simulink model "c00014M_harness"  (R2018a)
settings: Solver=ode3  StartTime=0.0  StopTime=10.0  RelTol=1e-3  EnableMultiTasking=on
undefined symbols (not defined in the file): b, DiscIntNeverNeededParam, J, K, L, PosMinimaW4, R, sigbuilder_block
(part 1 of 8)
settings Model: Creator=aarrieta  LastModifiedBy=umarkiegi
settings DataIOCC: LimitDataPoints=on  SaveFormat=Array
settings OptimizationCC: LifeSpan=inf
settings DebuggingCC: UnderspecifiedInitializationDetection=Classic  MergeDetectMultiDrivingBlocksExec=none  SolverPrmCheckMsg=warning  StateNameClashWarn=warning  SFUnexpectedBacktrackingDiag=warning  SFNoUnconditionalDefaultTransitionDiag=warning  SFExecutionAtInitializationDiag=none
settings HardwareCC: ProdBitPerPointer=32  ProdBitPerSizeT=32  ProdBitPerPtrDiffT=32  ProdLargestAtomicFloat=None  ProdIntDivRoundTo=Undefined  ProdEndianess=Unspecified  ProdWordSize=32  ProdHWDeviceType=32-bit Generic
settings ModelReferenceCC: PropagateSignalLabelsOutOfModel=off
settings CodeAppCC: StateflowObjectComments=on
settings GRTTargetCC: TargetLangStandard=C89/C90 (ANSI)  GeneratePreprocessorConditionals=Disable all
settings ConfigComp: CovMetricSettings=dw  CovHtmlReporting=on  CovSaveCumulativeToWorkspaceVar=on  CovSaveSingleToWorkspaceVar=on  CovExternalEMLEnable=off  DVMaxTestCaseSteps=20  DVTestSuiteOptimization=CombinedObjectives (Nonlinear Extended)  DVDetectFloatOverflow=off

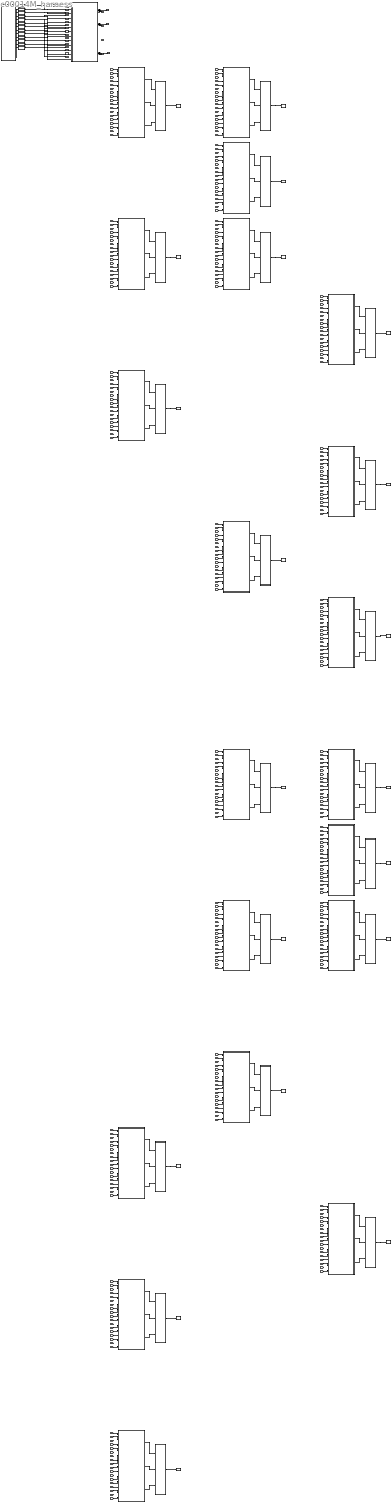
== system c00014M_harness ==
  CPSUT : Subsystem
  Eval : Subsystem
  Eval14 : Subsystem
  Eval16 : Subsystem
  Eval18 : Subsystem
  Eval2 : Subsystem
  Eval20 : Subsystem
  Eval21 : Subsystem
  Eval22 : Subsystem
  Eval26 : Subsystem
  Eval29 : Subsystem
  Eval31 : Subsystem
  Eval33 : Subsystem
  Eval4 : Subsystem
  Eval43 : Subsystem
  Eval45 : Subsystem
  Eval47 : Subsystem
  Eval49 : Subsystem
  Eval50 : Subsystem
  Eval51 : Subsystem
  Eval55 : Subsystem
  Inputs : Subsystem  Tag=STV Subsys  LoadFcn=sigbuilder_block('load');  StartFcn=sigbuilder_block('start');  StopFcn=sigbuilder_block('stop');  ClipboardFcn=sigbuilder_block('clipboard');  mask(Sigbuilder block){tuvar=[0:10]}
      mask init:
      | if ~strcmp(get_param(bdroot(gcb),'SimulationStatus'),'stopped'),tuvar = sigbuilder_block('maskInit'); end
      settings: CopyFcn=sigbuilder_block('copy');  DeleteFcn=sigbuilder_block('delete');  ModelCloseFcn=sigbuilder_block('modelClose');  PreSaveFcn=sigbuilder_block('preSave');  PauseFcn=sigbuilder_block('pause');  ContinueFcn=sigbuilder_block('continue');  NameChangeFcn=sigbuilder_block('namechange');  OpenFcn=sigbuilder_block('open');  CloseFcn=sigbuilder_block('close');
      mask Display: plot(0, 0, 100, 100,[2, 2, 32, 32, 2], [68, 8, 8, 68, 68],[32, 2], [38, 38], [32, 19, 2],[53, 60, 44], [32, 17, 17, 2],[16, 16, 31, 31]);txt = getActiveGroup(gcbh);text(2, 100, txt,'verticalAlignment', 'top');
  M001 : Subsystem
  M003 : Subsystem
  M005 : Subsystem
  M015 : Subsystem
  M017 : Subsystem
  M019 : Subsystem
  M021 : Subsystem
  M022 : Subsystem
  M023 : Subsystem
  M027 : Subsystem
  M030 : Subsystem
  M032 : Subsystem
  M034 : Subsystem
  M044 : Subsystem
  M046 : Subsystem
  M048 : Subsystem
  M050 : Subsystem
  M051 : Subsystem
  M052 : Subsystem
  M056 : Subsystem
  To Workspace : ToWorkspace  VariableName=mutant001  SampleTime=-1
  To Workspace14 : ToWorkspace  VariableName=mutant015  SampleTime=-1
  To Workspace16 : ToWorkspace  VariableName=mutant017  SampleTime=-1
  To Workspace18 : ToWorkspace  VariableName=mutant019  SampleTime=-1
  To Workspace2 : ToWorkspace  VariableName=mutant003  SampleTime=-1
  To Workspace20 : ToWorkspace  VariableName=mutant021  SampleTime=-1
  To Workspace21 : ToWorkspace  VariableName=mutant022  SampleTime=-1
  To Workspace22 : ToWorkspace  VariableName=mutant023  SampleTime=-1
  To Workspace26 : ToWorkspace  VariableName=mutant027  SampleTime=-1
  To Workspace29 : ToWorkspace  VariableName=mutant030  SampleTime=-1
  To Workspace31 : ToWorkspace  VariableName=mutant032  SampleTime=-1
  To Workspace33 : ToWorkspace  VariableName=mutant034  SampleTime=-1
  To Workspace4 : ToWorkspace  VariableName=mutant005  SampleTime=-1
  To Workspace43 : ToWorkspace  VariableName=mutant044  SampleTime=-1
  To Workspace45 : ToWorkspace  VariableName=mutant046  SampleTime=-1
  To Workspace47 : ToWorkspace  VariableName=mutant048  SampleTime=-1
  To Workspace49 : ToWorkspace  VariableName=mutant050  SampleTime=-1
  To Workspace50 : ToWorkspace  VariableName=mutant051  SampleTime=-1
  To Workspace51 : ToWorkspace  VariableName=mutant052  SampleTime=-1
  To Workspace55 : ToWorkspace  VariableName=mutant056  SampleTime=-1
  dtc_CW1C : DataTypeConversion
  dtc_CW2C : DataTypeConversion
  dtc_CW4C : DataTypeConversion
  dtc_DW1 : DataTypeConversion
  dtc_DW2 : DataTypeConversion
  dtc_DW4 : DataTypeConversion
  dtc_LD : DataTypeConversion
  dtc_O1 : DataTypeConversion
  dtc_O2 : DataTypeConversion
  dtc_O4 : DataTypeConversion
  dtc_P1W2 : DataTypeConversion
  dtc_P1W4 : DataTypeConversion
  dtc_P3W4 : DataTypeConversion
  W1Pos : Outport
  W2Pos : Outport  Port=2
  W4Pos : Outport  Port=3
  tag scope: out1=global, out2=global, out3=global, out4=global
  wires:
  CPSUT/2(W2Pos) -> [out2], W2Pos/1
  CPSUT/3(W4Pos) -> W4Pos/1, [out4]
  [in1] -> M001/1(DW1)
  [in2] -> M001/2(DW2)
  [in4] -> M001/3(DW4)
  [in5] -> M001/4(P1W2)
  [in8] -> M001/5(P3W4)
  [in9] -> M001/6(P1W4)
  [in10] -> M001/7(O1)
  [in11] -> M001/8(O2)
  [in13] -> M001/9(O4)
  [in14] -> M001/10(LD)
  [in15] -> M001/11(CW1C)
  [in16] -> M001/12(CW2C)
  [in18] -> M001/13(CW4C)
  CPSUT/1(W1Pos) -> [out1], W1Pos/1
  M001/1(W1Pos) -> Eval/1(In1)
  M001/2(W2Pos) -> Eval/2(In2)
  M001/3(W4Pos) -> Eval/3(In4)
  Eval/1(Out1) -> To Workspace/1
  [in1] -> M003/1(DW1)
  [in2] -> M003/2(DW2)
  [in4] -> M003/3(DW4)
  [in5] -> M003/4(P1W2)
  [in8] -> M003/5(P3W4)
  [in9] -> M003/6(P1W4)
  [in10] -> M003/7(O1)
  [in11] -> M003/8(O2)
  [in13] -> M003/9(O4)
  [in14] -> M003/10(LD)
  [in15] -> M003/11(CW1C)
  [in16] -> M003/12(CW2C)
  [in18] -> M003/13(CW4C)
  M003/1(W1Pos) -> Eval2/1(In1)
  M003/2(W2Pos) -> Eval2/2(In2)
  M003/3(W4Pos) -> Eval2/3(In4)
  Eval2/1(Out1) -> To Workspace2/1
  [in1] -> M005/1(DW1)
  [in2] -> M005/2(DW2)
  [in4] -> M005/3(DW4)
  [in5] -> M005/4(P1W2)
  [in8] -> M005/5(P3W4)
  [in9] -> M005/6(P1W4)
  [in10] -> M005/7(O1)
  [in11] -> M005/8(O2)
  [in13] -> M005/9(O4)
  [in14] -> M005/10(LD)
  [in15] -> M005/11(CW1C)
  [in16] -> M005/12(CW2C)
  [in18] -> M005/13(CW4C)
  M005/1(W1Pos) -> Eval4/1(In1)
  M005/2(W2Pos) -> Eval4/2(In2)
  M005/3(W4Pos) -> Eval4/3(In4)
  Eval4/1(Out1) -> To Workspace4/1
  [in1] -> M015/1(DW1)
  [in2] -> M015/2(DW2)
  [in4] -> M015/3(DW4)
  [in5] -> M015/4(P1W2)
  [in8] -> M015/5(P3W4)
  [in9] -> M015/6(P1W4)
  [in10] -> M015/7(O1)
  [in11] -> M015/8(O2)
  [in13] -> M015/9(O4)
  [in14] -> M015/10(LD)
  [in15] -> M015/11(CW1C)
  [in16] -> M015/12(CW2C)
  [in18] -> M015/13(CW4C)
  M015/1(W1Pos) -> Eval14/1(In1)
  M015/2(W2Pos) -> Eval14/2(In2)
  M015/3(W4Pos) -> Eval14/3(In4)
  Eval14/1(Out1) -> To Workspace14/1
  [in1] -> M017/1(DW1)
  [in2] -> M017/2(DW2)
  [in4] -> M017/3(DW4)
  [in5] -> M017/4(P1W2)
  [in8] -> M017/5(P3W4)
  [in9] -> M017/6(P1W4)
  [in10] -> M017/7(O1)
  [in11] -> M017/8(O2)
  [in13] -> M017/9(O4)
  [in14] -> M017/10(LD)
  [in15] -> M017/11(CW1C)
  [in16] -> M017/12(CW2C)
  [in18] -> M017/13(CW4C)
  M017/1(W1Pos) -> Eval16/1(In1)
  M017/2(W2Pos) -> Eval16/2(In2)
  M017/3(W4Pos) -> Eval16/3(In4)
  Eval16/1(Out1) -> To Workspace16/1
  [in1] -> M019/1(DW1)
  [in2] -> M019/2(DW2)
  [in4] -> M019/3(DW4)
  [in5] -> M019/4(P1W2)
  [in8] -> M019/5(P3W4)
  [in9] -> M019/6(P1W4)
  [in10] -> M019/7(O1)
  [in11] -> M019/8(O2)
  [in13] -> M019/9(O4)
  [in14] -> M019/10(LD)
  [in15] -> M019/11(CW1C)
  [in16] -> M019/12(CW2C)
  [in18] -> M019/13(CW4C)
  M019/1(W1Pos) -> Eval18/1(In1)
  M019/2(W2Pos) -> Eval18/2(In2)
  M019/3(W4Pos) -> Eval18/3(In4)
  Eval18/1(Out1) -> To Workspace18/1
  [in1] -> M021/1(DW1)
  [in2] -> M021/2(DW2)
  [in4] -> M021/3(DW4)
  [in5] -> M021/4(P1W2)
  [in8] -> M021/5(P3W4)
  [in9] -> M021/6(P1W4)
  [in10] -> M021/7(O1)
  [in11] -> M021/8(O2)
  [in13] -> M021/9(O4)
  [in14] -> M021/10(LD)
  [in15] -> M021/11(CW1C)
  [in16] -> M021/12(CW2C)
  [in18] -> M021/13(CW4C)
  M021/1(W1Pos) -> Eval20/1(In1)
  M021/2(W2Pos) -> Eval20/2(In2)
  M021/3(W4Pos) -> Eval20/3(In4)
  Eval20/1(Out1) -> To Workspace20/1
  [in1] -> M022/1(DW1)
  [in2] -> M022/2(DW2)
  [in4] -> M022/3(DW4)
  [in5] -> M022/4(P1W2)
  [in8] -> M022/5(P3W4)
  [in9] -> M022/6(P1W4)
  [in10] -> M022/7(O1)
  [in11] -> M022/8(O2)
  [in13] -> M022/9(O4)
  [in14] -> M022/10(LD)
  [in15] -> M022/11(CW1C)
  [in16] -> M022/12(CW2C)
  [in18] -> M022/13(CW4C)
  M022/1(W1Pos) -> Eval21/1(In1)
  M022/2(W2Pos) -> Eval21/2(In2)
  M022/3(W4Pos) -> Eval21/3(In4)
  Eval21/1(Out1) -> To Workspace21/1
  [in1] -> M023/1(DW1)
  [in2] -> M023/2(DW2)
  [in4] -> M023/3(DW4)
  [in5] -> M023/4(P1W2)
  [in8] -> M023/5(P3W4)
  [in9] -> M023/6(P1W4)
  [in10] -> M023/7(O1)
  [in11] -> M023/8(O2)
  [in13] -> M023/9(O4)
  [in14] -> M023/10(LD)
  [in15] -> M023/11(CW1C)
  [in16] -> M023/12(CW2C)
  [in18] -> M023/13(CW4C)
  M023/1(W1Pos) -> Eval22/1(In1)
  M023/2(W2Pos) -> Eval22/2(In2)
  M023/3(W4Pos) -> Eval22/3(In4)
  Eval22/1(Out1) -> To Workspace22/1
  [in1] -> M027/1(DW1)
  [in2] -> M027/2(DW2)
  [in4] -> M027/3(DW4)
  [in5] -> M027/4(P1W2)
  [in8] -> M027/5(P3W4)
  [in9] -> M027/6(P1W4)
  [in10] -> M027/7(O1)
  [in11] -> M027/8(O2)
  [in13] -> M027/9(O4)
  [in14] -> M027/10(LD)
  [in15] -> M027/11(CW1C)
  [in16] -> M027/12(CW2C)
  [in18] -> M027/13(CW4C)
  M027/1(W1Pos) -> Eval26/1(In1)
  M027/2(W2Pos) -> Eval26/2(In2)
  M027/3(W4Pos) -> Eval26/3(In4)
  Eval26/1(Out1) -> To Workspace26/1
  [in1] -> M030/1(DW1)
  [in2] -> M030/2(DW2)
  [in4] -> M030/3(DW4)
  [in5] -> M030/4(P1W2)
  [in8] -> M030/5(P3W4)
  [in9] -> M030/6(P1W4)
  [in10] -> M030/7(O1)
  [in11] -> M030/8(O2)
  [in13] -> M030/9(O4)
  [in14] -> M030/10(LD)
  [in15] -> M030/11(CW1C)
  [in16] -> M030/12(CW2C)
  [in18] -> M030/13(CW4C)
  M030/1(W1Pos) -> Eval29/1(In1)
  M030/2(W2Pos) -> Eval29/2(In2)
  M030/3(W4Pos) -> Eval29/3(In4)
  Eval29/1(Out1) -> To Workspace29/1
  [in1] -> M032/1(DW1)
  [in2] -> M032/2(DW2)
  [in4] -> M032/3(DW4)
  [in5] -> M032/4(P1W2)
  [in8] -> M032/5(P3W4)
  [in9] -> M032/6(P1W4)
  [in10] -> M032/7(O1)
  [in11] -> M032/8(O2)
  [in13] -> M032/9(O4)
  [in14] -> M032/10(LD)
  [in15] -> M032/11(CW1C)
  [in16] -> M032/12(CW2C)
  [in18] -> M032/13(CW4C)
  M032/1(W1Pos) -> Eval31/1(In1)
  M032/2(W2Pos) -> Eval31/2(In2)
  M032/3(W4Pos) -> Eval31/3(In4)
  Eval31/1(Out1) -> To Workspace31/1
  [in1] -> M034/1(DW1)
  [in2] -> M034/2(DW2)
  [in4] -> M034/3(DW4)
  [in5] -> M034/4(P1W2)
  [in8] -> M034/5(P3W4)
  [in9] -> M034/6(P1W4)
  [in10] -> M034/7(O1)
  [in11] -> M034/8(O2)
  [in13] -> M034/9(O4)
  [in14] -> M034/10(LD)
  [in15] -> M034/11(CW1C)
  [in16] -> M034/12(CW2C)
  [in18] -> M034/13(CW4C)
  M034/1(W1Pos) -> Eval33/1(In1)
  M034/2(W2Pos) -> Eval33/2(In2)
  M034/3(W4Pos) -> Eval33/3(In4)
  Eval33/1(Out1) -> To Workspace33/1
  [in1] -> M044/1(DW1)
  [in2] -> M044/2(DW2)
  [in4] -> M044/3(DW4)
  [in5] -> M044/4(P1W2)
  [in8] -> M044/5(P3W4)
  [in9] -> M044/6(P1W4)
  [in10] -> M044/7(O1)
  [in11] -> M044/8(O2)
  [in13] -> M044/9(O4)
  [in14] -> M044/10(LD)
  [in15] -> M044/11(CW1C)
  [in16] -> M044/12(CW2C)
  [in18] -> M044/13(CW4C)
  M044/1(W1Pos) -> Eval43/1(In1)
  M044/2(W2Pos) -> Eval43/2(In2)
  M044/3(W4Pos) -> Eval43/3(In4)
  Eval43/1(Out1) -> To Workspace43/1
  [in1] -> M046/1(DW1)
  [in2] -> M046/2(DW2)
  [in4] -> M046/3(DW4)
  [in5] -> M046/4(P1W2)
  [in8] -> M046/5(P3W4)
  [in9] -> M046/6(P1W4)
  [in10] -> M046/7(O1)
  [in11] -> M046/8(O2)
  [in13] -> M046/9(O4)
  [in14] -> M046/10(LD)
  [in15] -> M046/11(CW1C)
  [in16] -> M046/12(CW2C)
  [in18] -> M046/13(CW4C)
  M046/1(W1Pos) -> Eval45/1(In1)
  M046/2(W2Pos) -> Eval45/2(In2)
  M046/3(W4Pos) -> Eval45/3(In4)
  Eval45/1(Out1) -> To Workspace45/1
  [in1] -> M048/1(DW1)
  [in2] -> M048/2(DW2)
  [in4] -> M048/3(DW4)
  [in5] -> M048/4(P1W2)
  [in8] -> M048/5(P3W4)
  [in9] -> M048/6(P1W4)
  [in10] -> M048/7(O1)
  [in11] -> M048/8(O2)
  [in13] -> M048/9(O4)
  [in14] -> M048/10(LD)
  [in15] -> M048/11(CW1C)
  [in16] -> M048/12(CW2C)
  [in18] -> M048/13(CW4C)
  M048/1(W1Pos) -> Eval47/1(In1)
  M048/2(W2Pos) -> Eval47/2(In2)
  M048/3(W4Pos) -> Eval47/3(In4)
  Eval47/1(Out1) -> To Workspace47/1
  [in1] -> M050/1(DW1)
  [in2] -> M050/2(DW2)
  [in4] -> M050/3(DW4)
  [in5] -> M050/4(P1W2)
  [in8] -> M050/5(P3W4)
  [in9] -> M050/6(P1W4)
  [in10] -> M050/7(O1)
  [in11] -> M050/8(O2)
  [in13] -> M050/9(O4)
  [in14] -> M050/10(LD)
  [in15] -> M050/11(CW1C)
  [in16] -> M050/12(CW2C)
  [in18] -> M050/13(CW4C)
  M050/1(W1Pos) -> Eval49/1(In1)
  M050/2(W2Pos) -> Eval49/2(In2)
  M050/3(W4Pos) -> Eval49/3(In4)
  Eval49/1(Out1) -> To Workspace49/1
  [in1] -> M051/1(DW1)
  [in2] -> M051/2(DW2)
  [in4] -> M051/3(DW4)
  [in5] -> M051/4(P1W2)
  [in8] -> M051/5(P3W4)
  [in9] -> M051/6(P1W4)
  [in10] -> M051/7(O1)
  [in11] -> M051/8(O2)
  [in13] -> M051/9(O4)
  [in14] -> M051/10(LD)
  [in15] -> M051/11(CW1C)
  [in16] -> M051/12(CW2C)
  [in18] -> M051/13(CW4C)
  M051/1(W1Pos) -> Eval50/1(In1)
  M051/2(W2Pos) -> Eval50/2(In2)
  M051/3(W4Pos) -> Eval50/3(In4)
  Eval50/1(Out1) -> To Workspace50/1
  [in1] -> M052/1(DW1)
  [in2] -> M052/2(DW2)
  [in4] -> M052/3(DW4)
  [in5] -> M052/4(P1W2)
  [in8] -> M052/5(P3W4)
  [in9] -> M052/6(P1W4)
  [in10] -> M052/7(O1)
  [in11] -> M052/8(O2)
  [in13] -> M052/9(O4)
  [in14] -> M052/10(LD)
  [in15] -> M052/11(CW1C)
  [in16] -> M052/12(CW2C)
  [in18] -> M052/13(CW4C)
  M052/1(W1Pos) -> Eval51/1(In1)
  M052/2(W2Pos) -> Eval51/2(In2)
  M052/3(W4Pos) -> Eval51/3(In4)
  Eval51/1(Out1) -> To Workspace51/1
  [in1] -> M056/1(DW1)
  [in2] -> M056/2(DW2)
  [in4] -> M056/3(DW4)
  [in5] -> M056/4(P1W2)
  [in8] -> M056/5(P3W4)
  [in9] -> M056/6(P1W4)
  [in10] -> M056/7(O1)
  [in11] -> M056/8(O2)
  [in13] -> M056/9(O4)
  [in14] -> M056/10(LD)
  [in15] -> M056/11(CW1C)
  [in16] -> M056/12(CW2C)
  [in18] -> M056/13(CW4C)
  M056/1(W1Pos) -> Eval55/1(In1)
  M056/2(W2Pos) -> Eval55/2(In2)
  M056/3(W4Pos) -> Eval55/3(In4)
  Eval55/1(Out1) -> To Workspace55/1
  Inputs/1(DW1) -> dtc_DW1/1
  dtc_DW1/1 -> CPSUT/1(DW1), [in1]
  Inputs/2(DW2) -> dtc_DW2/1
  dtc_DW2/1 -> CPSUT/2(DW2), [in2]
  Inputs/3(DW4) -> dtc_DW4/1
  dtc_DW4/1 -> CPSUT/3(DW4), [in4]
  Inputs/4(P1W2) -> dtc_P1W2/1
  dtc_P1W2/1 -> CPSUT/4(P1W2), [in5]
  Inputs/5(P3W4) -> dtc_P3W4/1
  dtc_P3W4/1 -> CPSUT/5(P3W4), [in8]
  Inputs/6(P1W4) -> dtc_P1W4/1
  dtc_P1W4/1 -> CPSUT/6(P1W4), [in9]
  Inputs/7(O1) -> dtc_O1/1
  dtc_O1/1 -> CPSUT/7(O1), [in10]
  Inputs/8(O2) -> dtc_O2/1
  dtc_O2/1 -> CPSUT/8(O2), [in11]
  Inputs/9(O4) -> dtc_O4/1
  dtc_O4/1 -> CPSUT/9(O4), [in13]
  Inputs/10(LD) -> dtc_LD/1
  dtc_LD/1 -> CPSUT/10(LD), [in14]
  Inputs/11(CW1C) -> dtc_CW1C/1
  dtc_CW1C/1 -> CPSUT/11(CW1C), [in15]
  Inputs/12(CW2C) -> dtc_CW2C/1
  dtc_CW2C/1 -> CPSUT/12(CW2C), [in16]
  Inputs/13(CW4C) -> dtc_CW4C/1
  dtc_CW4C/1 -> CPSUT/13(CW4C), [in18]

== system c00014M_harness/CPSUT ==
  DW1 : Inport  OutMin=0  OutMax=4  OutDataTypeStr=int8
  DW2 : Inport  Port=2  OutMin=0  OutMax=4  OutDataTypeStr=int8
  DW4 : Inport  Port=3  OutMin=0  OutMax=4  OutDataTypeStr=int8
  P1W2 : Inport  Port=4  OutMin=0  OutMax=4  OutDataTypeStr=int8
  P3W4 : Inport  Port=5  OutMin=0  OutMax=4  OutDataTypeStr=int8
  P1W4 : Inport  Port=6  OutMin=0  OutMax=4  OutDataTypeStr=int8
  O1 : Inport  Port=7  OutDataTypeStr=boolean
  O2 : Inport  Port=8  OutDataTypeStr=boolean
  O4 : Inport  Port=9  OutDataTypeStr=boolean
  LD : Inport  Port=10  OutDataTypeStr=boolean
  CW1C : Inport  Port=11  OutMin=0  OutMax=4  OutDataTypeStr=int8
  CW2C : Inport  Port=12  OutMin=0  OutMax=4  OutDataTypeStr=int8
  CW4C : Inport  Port=13  OutMin=0  OutMax=4  OutDataTypeStr=int8
  Cyber : Subsystem
  M : Memory
  M1 : Memory
  M3 : Memory
  Physical : Subsystem
  S1 : Subsystem
  S2 : Subsystem
  S4 : Subsystem
  W1Pos : Outport
  W2Pos : Outport  Port=2
  W4Pos : Outport  Port=3
  wires:
  M3/1 -> Cyber/3(PosW4)
  S1/1(SensorOut) -> M/1
  CW2C/1 -> Cyber/15(CW2C)
  CW4C/1 -> Cyber/16(CW4C)
  Physical/1(W1) -> W1Pos/1, S1/1(PhyMeasure)
  O4/1 -> Cyber/12(OW4)
  O2/1 -> Cyber/11(OW2)
  LD/1 -> Cyber/13(LD)
  O1/1 -> Cyber/10(OW1)
  Cyber/1(W1) -> Physical/1(InW1)
  Cyber/2(W2) -> Physical/2(InW2)
  P1W2/1 -> Cyber/7(P1W2)
  P1W4/1 -> Cyber/9(P1W4)
  CW1C/1 -> Cyber/14(CW1C)
  S4/1(SensorOut) -> M3/1
  M1/1 -> Cyber/2(PosW2)
  M/1 -> Cyber/1(PosW1)
  DW1/1 -> Cyber/4(DW1)
  Physical/2(W2) -> W2Pos/1, S2/1(PhyMeasure)
  S2/1(SensorOut) -> M1/1
  P3W4/1 -> Cyber/8(P3W4)
  DW2/1 -> Cyber/5(DW2)
  Physical/3(W4) -> W4Pos/1, S4/1(PhyMeasure)
  DW4/1 -> Cyber/6(DW4)
  Cyber/3(W4) -> Physical/3(InW4)

== system c00014M_harness/Eval ==
  In1 : Inport
  In2 : Inport  Port=2
  In4 : Inport  Port=3
  Constant3 : Constant
  Data Type Conversion : DataTypeConversion
  Data Type Conversion1 : DataTypeConversion
  Data Type Conversion3 : DataTypeConversion
  Memory1 : Memory  InitialCondition=1
  Memory2 : Memory  InitialCondition=1
  Memory4 : Memory  InitialCondition=1
  MinMax : MinMax  Inputs=4
  MinMax1 : MinMax  Inputs=2
  MinMax2 : MinMax  Inputs=2
  MinMax4 : MinMax  Inputs=2
  ROOut1 : RelationalOperator  Operator===  OutDataTypeStr=boolean  RndMeth=Simplest
  ROOut2 : RelationalOperator  Operator===  OutDataTypeStr=boolean  RndMeth=Simplest
  ROOut4 : RelationalOperator  Operator===  OutDataTypeStr=boolean  RndMeth=Simplest
  Out1 : Outport
  wires:
  MinMax/1 -> Out1/1
  [out1] -> ROOut1/2
  In2/1 -> ROOut2/1
  In1/1 -> ROOut1/1
  [out2] -> ROOut2/2
  In4/1 -> ROOut4/1
  [out4] -> ROOut4/2
  Memory1/1 -> MinMax1/2
  MinMax4/1 -> MinMax/4, Memory4/1
  ROOut2/1 -> Data Type Conversion1/1
  Memory4/1 -> MinMax4/2
  Memory2/1 -> MinMax2/2
  ROOut1/1 -> Data Type Conversion/1
  MinMax2/1 -> MinMax/2, Memory2/1
  ROOut4/1 -> Data Type Conversion3/1
  MinMax1/1 -> MinMax/1, Memory1/1
  Data Type Conversion/1 -> MinMax1/1
  Data Type Conversion1/1 -> MinMax2/1
  Data Type Conversion3/1 -> MinMax4/1
  Constant3/1 -> MinMax/3

== system c00014M_harness/Eval14 ==
  In1 : Inport
  In2 : Inport  Port=2
  In4 : Inport  Port=3
  Constant3 : Constant
  Data Type Conversion : DataTypeConversion
  Data Type Conversion1 : DataTypeConversion
  Data Type Conversion3 : DataTypeConversion
  Memory1 : Memory  InitialCondition=1
  Memory2 : Memory  InitialCondition=1
  Memory4 : Memory  InitialCondition=1
  MinMax : MinMax  Inputs=4
  MinMax1 : MinMax  Inputs=2
  MinMax2 : MinMax  Inputs=2
  MinMax4 : MinMax  Inputs=2
  ROOut1 : RelationalOperator  Operator===  OutDataTypeStr=boolean  RndMeth=Simplest
  ROOut2 : RelationalOperator  Operator===  OutDataTypeStr=boolean  RndMeth=Simplest
  ROOut4 : RelationalOperator  Operator===  OutDataTypeStr=boolean  RndMeth=Simplest
  Out1 : Outport
  wires:
  Data Type Conversion3/1 -> MinMax4/1
  Data Type Conversion1/1 -> MinMax2/1
  Data Type Conversion/1 -> MinMax1/1
  MinMax1/1 -> Memory1/1, MinMax/1
  ROOut4/1 -> Data Type Conversion3/1
  MinMax2/1 -> Memory2/1, MinMax/2
  ROOut1/1 -> Data Type Conversion/1
  Memory2/1 -> MinMax2/2
  Memory4/1 -> MinMax4/2
  ROOut2/1 -> Data Type Conversion1/1
  MinMax4/1 -> Memory4/1, MinMax/4
  Memory1/1 -> MinMax1/2
  [out4] -> ROOut4/2
  In4/1 -> ROOut4/1
  [out2] -> ROOut2/2
  In1/1 -> ROOut1/1
  In2/1 -> ROOut2/1
  [out1] -> ROOut1/2
  MinMax/1 -> Out1/1
  Constant3/1 -> MinMax/3

== system c00014M_harness/Eval16 ==
  In1 : Inport
  In2 : Inport  Port=2
  In4 : Inport  Port=3
  Constant3 : Constant
  Data Type Conversion : DataTypeConversion
  Data Type Conversion1 : DataTypeConversion
  Data Type Conversion3 : DataTypeConversion
  Memory1 : Memory  InitialCondition=1
  Memory2 : Memory  InitialCondition=1
  Memory4 : Memory  InitialCondition=1
  MinMax : MinMax  Inputs=4
  MinMax1 : MinMax  Inputs=2
  MinMax2 : MinMax  Inputs=2
  MinMax4 : MinMax  Inputs=2
  ROOut1 : RelationalOperator  Operator===  OutDataTypeStr=boolean  RndMeth=Simplest
  ROOut2 : RelationalOperator  Operator===  OutDataTypeStr=boolean  RndMeth=Simplest
  ROOut4 : RelationalOperator  Operator===  OutDataTypeStr=boolean  RndMeth=Simplest
  Out1 : Outport
  wires:
  Data Type Conversion3/1 -> MinMax4/1
  Data Type Conversion1/1 -> MinMax2/1
  Data Type Conversion/1 -> MinMax1/1
  MinMax1/1 -> Memory1/1, MinMax/1
  ROOut4/1 -> Data Type Conversion3/1
  MinMax2/1 -> Memory2/1, MinMax/2
  ROOut1/1 -> Data Type Conversion/1
  Memory2/1 -> MinMax2/2
  Memory4/1 -> MinMax4/2
  ROOut2/1 -> Data Type Conversion1/1
  MinMax4/1 -> Memory4/1, MinMax/4
  Memory1/1 -> MinMax1/2
  [out4] -> ROOut4/2
  In4/1 -> ROOut4/1
  [out2] -> ROOut2/2
  In1/1 -> ROOut1/1
  In2/1 -> ROOut2/1
  [out1] -> ROOut1/2
  MinMax/1 -> Out1/1
  Constant3/1 -> MinMax/3

== system c00014M_harness/Eval18 ==
  In1 : Inport
  In2 : Inport  Port=2
  In4 : Inport  Port=3
  Constant3 : Constant
  Data Type Conversion : DataTypeConversion
  Data Type Conversion1 : DataTypeConversion
  Data Type Conversion3 : DataTypeConversion
  Memory1 : Memory  InitialCondition=1
  Memory2 : Memory  InitialCondition=1
  Memory4 : Memory  InitialCondition=1
  MinMax : MinMax  Inputs=4
  MinMax1 : MinMax  Inputs=2
  MinMax2 : MinMax  Inputs=2
  MinMax4 : MinMax  Inputs=2
  ROOut1 : RelationalOperator  Operator===  OutDataTypeStr=boolean  RndMeth=Simplest
  ROOut2 : RelationalOperator  Operator===  OutDataTypeStr=boolean  RndMeth=Simplest
  ROOut4 : RelationalOperator  Operator===  OutDataTypeStr=boolean  RndMeth=Simplest
  Out1 : Outport
  wires:
  Data Type Conversion3/1 -> MinMax4/1
  Data Type Conversion1/1 -> MinMax2/1
  Data Type Conversion/1 -> MinMax1/1
  MinMax1/1 -> Memory1/1, MinMax/1
  ROOut4/1 -> Data Type Conversion3/1
  MinMax2/1 -> Memory2/1, MinMax/2
  ROOut1/1 -> Data Type Conversion/1
  Memory2/1 -> MinMax2/2
  Memory4/1 -> MinMax4/2
  ROOut2/1 -> Data Type Conversion1/1
  MinMax4/1 -> Memory4/1, MinMax/4
  Memory1/1 -> MinMax1/2
  [out4] -> ROOut4/2
  In4/1 -> ROOut4/1
  [out2] -> ROOut2/2
  In1/1 -> ROOut1/1
  In2/1 -> ROOut2/1
  [out1] -> ROOut1/2
  MinMax/1 -> Out1/1
  Constant3/1 -> MinMax/3

== system c00014M_harness/Eval2 ==
  In1 : Inport
  In2 : Inport  Port=2
  In4 : Inport  Port=3
  Constant3 : Constant
  Data Type Conversion : DataTypeConversion
  Data Type Conversion1 : DataTypeConversion
  Data Type Conversion3 : DataTypeConversion
  Memory1 : Memory  InitialCondition=1
  Memory2 : Memory  InitialCondition=1
  Memory4 : Memory  InitialCondition=1
  MinMax : MinMax  Inputs=4
  MinMax1 : MinMax  Inputs=2
  MinMax2 : MinMax  Inputs=2
  MinMax4 : MinMax  Inputs=2
  ROOut1 : RelationalOperator  Operator===  OutDataTypeStr=boolean  RndMeth=Simplest
  ROOut2 : RelationalOperator  Operator===  OutDataTypeStr=boolean  RndMeth=Simplest
  ROOut4 : RelationalOperator  Operator===  OutDataTypeStr=boolean  RndMeth=Simplest
  Out1 : Outport
  wires:
  Data Type Conversion3/1 -> MinMax4/1
  Data Type Conversion1/1 -> MinMax2/1
  Data Type Conversion/1 -> MinMax1/1
  MinMax1/1 -> Memory1/1, MinMax/1
  ROOut4/1 -> Data Type Conversion3/1
  MinMax2/1 -> Memory2/1, MinMax/2
  ROOut1/1 -> Data Type Conversion/1
  Memory2/1 -> MinMax2/2
  Memory4/1 -> MinMax4/2
  ROOut2/1 -> Data Type Conversion1/1
  MinMax4/1 -> Memory4/1, MinMax/4
  Memory1/1 -> MinMax1/2
  [out4] -> ROOut4/2
  In4/1 -> ROOut4/1
  [out2] -> ROOut2/2
  In1/1 -> ROOut1/1
  In2/1 -> ROOut2/1
  [out1] -> ROOut1/2
  MinMax/1 -> Out1/1
  Constant3/1 -> MinMax/3

== system c00014M_harness/Eval20 ==
  In1 : Inport
  In2 : Inport  Port=2
  In4 : Inport  Port=3
  Constant3 : Constant
  Data Type Conversion : DataTypeConversion
  Data Type Conversion1 : DataTypeConversion
  Data Type Conversion3 : DataTypeConversion
  Memory1 : Memory  InitialCondition=1
  Memory2 : Memory  InitialCondition=1
  Memory4 : Memory  InitialCondition=1
  MinMax : MinMax  Inputs=4
  MinMax1 : MinMax  Inputs=2
  MinMax2 : MinMax  Inputs=2
  MinMax4 : MinMax  Inputs=2
  ROOut1 : RelationalOperator  Operator===  OutDataTypeStr=boolean  RndMeth=Simplest
  ROOut2 : RelationalOperator  Operator===  OutDataTypeStr=boolean  RndMeth=Simplest
  ROOut4 : RelationalOperator  Operator===  OutDataTypeStr=boolean  RndMeth=Simplest
  Out1 : Outport
  wires:
  Data Type Conversion3/1 -> MinMax4/1
  Data Type Conversion1/1 -> MinMax2/1
  Data Type Conversion/1 -> MinMax1/1
  MinMax1/1 -> Memory1/1, MinMax/1
  ROOut4/1 -> Data Type Conversion3/1
  MinMax2/1 -> Memory2/1, MinMax/2
  ROOut1/1 -> Data Type Conversion/1
  Memory2/1 -> MinMax2/2
  Memory4/1 -> MinMax4/2
  ROOut2/1 -> Data Type Conversion1/1
  MinMax4/1 -> Memory4/1, MinMax/4
  Memory1/1 -> MinMax1/2
  [out4] -> ROOut4/2
  In4/1 -> ROOut4/1
  [out2] -> ROOut2/2
  In1/1 -> ROOut1/1
  In2/1 -> ROOut2/1
  [out1] -> ROOut1/2
  MinMax/1 -> Out1/1
  Constant3/1 -> MinMax/3

== system c00014M_harness/Eval21 ==
  In1 : Inport
  In2 : Inport  Port=2
  In4 : Inport  Port=3
  Constant3 : Constant
  Data Type Conversion : DataTypeConversion
  Data Type Conversion1 : DataTypeConversion
  Data Type Conversion3 : DataTypeConversion
  Memory1 : Memory  InitialCondition=1
  Memory2 : Memory  InitialCondition=1
  Memory4 : Memory  InitialCondition=1
  MinMax : MinMax  Inputs=4
  MinMax1 : MinMax  Inputs=2
  MinMax2 : MinMax  Inputs=2
  MinMax4 : MinMax  Inputs=2
  ROOut1 : RelationalOperator  Operator===  OutDataTypeStr=boolean  RndMeth=Simplest
  ROOut2 : RelationalOperator  Operator===  OutDataTypeStr=boolean  RndMeth=Simplest
  ROOut4 : RelationalOperator  Operator===  OutDataTypeStr=boolean  RndMeth=Simplest
  Out1 : Outport
  wires:
  Data Type Conversion3/1 -> MinMax4/1
  Data Type Conversion1/1 -> MinMax2/1
  Data Type Conversion/1 -> MinMax1/1
  MinMax1/1 -> Memory1/1, MinMax/1
  ROOut4/1 -> Data Type Conversion3/1
  MinMax2/1 -> Memory2/1, MinMax/2
  ROOut1/1 -> Data Type Conversion/1
  Memory2/1 -> MinMax2/2
  Memory4/1 -> MinMax4/2
  ROOut2/1 -> Data Type Conversion1/1
  MinMax4/1 -> Memory4/1, MinMax/4
  Memory1/1 -> MinMax1/2
  [out4] -> ROOut4/2
  In4/1 -> ROOut4/1
  [out2] -> ROOut2/2
  In1/1 -> ROOut1/1
  In2/1 -> ROOut2/1
  [out1] -> ROOut1/2
  MinMax/1 -> Out1/1
  Constant3/1 -> MinMax/3

== system c00014M_harness/Eval22 ==
  In1 : Inport
  In2 : Inport  Port=2
  In4 : Inport  Port=3
  Constant3 : Constant
  Data Type Conversion : DataTypeConversion
  Data Type Conversion1 : DataTypeConversion
  Data Type Conversion3 : DataTypeConversion
  Memory1 : Memory  InitialCondition=1
  Memory2 : Memory  InitialCondition=1
  Memory4 : Memory  InitialCondition=1
  MinMax : MinMax  Inputs=4
  MinMax1 : MinMax  Inputs=2
  MinMax2 : MinMax  Inputs=2
  MinMax4 : MinMax  Inputs=2
  ROOut1 : RelationalOperator  Operator===  OutDataTypeStr=boolean  RndMeth=Simplest
  ROOut2 : RelationalOperator  Operator===  OutDataTypeStr=boolean  RndMeth=Simplest
  ROOut4 : RelationalOperator  Operator===  OutDataTypeStr=boolean  RndMeth=Simplest
  Out1 : Outport
  wires:
  Data Type Conversion3/1 -> MinMax4/1
  Data Type Conversion1/1 -> MinMax2/1
  Data Type Conversion/1 -> MinMax1/1
  MinMax1/1 -> Memory1/1, MinMax/1
  ROOut4/1 -> Data Type Conversion3/1
  MinMax2/1 -> Memory2/1, MinMax/2
  ROOut1/1 -> Data Type Conversion/1
  Memory2/1 -> MinMax2/2
  Memory4/1 -> MinMax4/2
  ROOut2/1 -> Data Type Conversion1/1
  MinMax4/1 -> Memory4/1, MinMax/4
  Memory1/1 -> MinMax1/2
  [out4] -> ROOut4/2
  In4/1 -> ROOut4/1
  [out2] -> ROOut2/2
  In1/1 -> ROOut1/1
  In2/1 -> ROOut2/1
  [out1] -> ROOut1/2
  MinMax/1 -> Out1/1
  Constant3/1 -> MinMax/3

== system c00014M_harness/Eval26 ==
  In1 : Inport
  In2 : Inport  Port=2
  In4 : Inport  Port=3
  Constant3 : Constant
  Data Type Conversion : DataTypeConversion
  Data Type Conversion1 : DataTypeConversion
  Data Type Conversion3 : DataTypeConversion
  Memory1 : Memory  InitialCondition=1
  Memory2 : Memory  InitialCondition=1
  Memory4 : Memory  InitialCondition=1
  MinMax : MinMax  Inputs=4
  MinMax1 : MinMax  Inputs=2
  MinMax2 : MinMax  Inputs=2
  MinMax4 : MinMax  Inputs=2
  ROOut1 : RelationalOperator  Operator===  OutDataTypeStr=boolean  RndMeth=Simplest
  ROOut2 : RelationalOperator  Operator===  OutDataTypeStr=boolean  RndMeth=Simplest
  ROOut4 : RelationalOperator  Operator===  OutDataTypeStr=boolean  RndMeth=Simplest
  Out1 : Outport
  wires:
  Data Type Conversion3/1 -> MinMax4/1
  Data Type Conversion1/1 -> MinMax2/1
  Data Type Conversion/1 -> MinMax1/1
  MinMax1/1 -> Memory1/1, MinMax/1
  ROOut4/1 -> Data Type Conversion3/1
  MinMax2/1 -> Memory2/1, MinMax/2
  ROOut1/1 -> Data Type Conversion/1
  Memory2/1 -> MinMax2/2
  Memory4/1 -> MinMax4/2
  ROOut2/1 -> Data Type Conversion1/1
  MinMax4/1 -> Memory4/1, MinMax/4
  Memory1/1 -> MinMax1/2
  [out4] -> ROOut4/2
  In4/1 -> ROOut4/1
  [out2] -> ROOut2/2
  In1/1 -> ROOut1/1
  In2/1 -> ROOut2/1
  [out1] -> ROOut1/2
  MinMax/1 -> Out1/1
  Constant3/1 -> MinMax/3

== system c00014M_harness/Eval29 ==
  In1 : Inport
  In2 : Inport  Port=2
  In4 : Inport  Port=3
  Constant3 : Constant
  Data Type Conversion : DataTypeConversion
  Data Type Conversion1 : DataTypeConversion
  Data Type Conversion3 : DataTypeConversion
  Memory1 : Memory  InitialCondition=1
  Memory2 : Memory  InitialCondition=1
  Memory4 : Memory  InitialCondition=1
  MinMax : MinMax  Inputs=4
  MinMax1 : MinMax  Inputs=2
  MinMax2 : MinMax  Inputs=2
  MinMax4 : MinMax  Inputs=2
  ROOut1 : RelationalOperator  Operator===  OutDataTypeStr=boolean  RndMeth=Simplest
  ROOut2 : RelationalOperator  Operator===  OutDataTypeStr=boolean  RndMeth=Simplest
  ROOut4 : RelationalOperator  Operator===  OutDataTypeStr=boolean  RndMeth=Simplest
  Out1 : Outport
  wires:
  Data Type Conversion3/1 -> MinMax4/1
  Data Type Conversion1/1 -> MinMax2/1
  Data Type Conversion/1 -> MinMax1/1
  MinMax1/1 -> Memory1/1, MinMax/1
  ROOut4/1 -> Data Type Conversion3/1
  MinMax2/1 -> Memory2/1, MinMax/2
  ROOut1/1 -> Data Type Conversion/1
  Memory2/1 -> MinMax2/2
  Memory4/1 -> MinMax4/2
  ROOut2/1 -> Data Type Conversion1/1
  MinMax4/1 -> Memory4/1, MinMax/4
  Memory1/1 -> MinMax1/2
  [out4] -> ROOut4/2
  In4/1 -> ROOut4/1
  [out2] -> ROOut2/2
  In1/1 -> ROOut1/1
  In2/1 -> ROOut2/1
  [out1] -> ROOut1/2
  MinMax/1 -> Out1/1
  Constant3/1 -> MinMax/3

== system c00014M_harness/Eval31 ==
  In1 : Inport
  In2 : Inport  Port=2
  In4 : Inport  Port=3
  Constant3 : Constant
  Data Type Conversion : DataTypeConversion
  Data Type Conversion1 : DataTypeConversion
  Data Type Conversion3 : DataTypeConversion
  Memory1 : Memory  InitialCondition=1
  Memory2 : Memory  InitialCondition=1
  Memory4 : Memory  InitialCondition=1
  MinMax : MinMax  Inputs=4
  MinMax1 : MinMax  Inputs=2
  MinMax2 : MinMax  Inputs=2
  MinMax4 : MinMax  Inputs=2
  ROOut1 : RelationalOperator  Operator===  OutDataTypeStr=boolean  RndMeth=Simplest
  ROOut2 : RelationalOperator  Operator===  OutDataTypeStr=boolean  RndMeth=Simplest
  ROOut4 : RelationalOperator  Operator===  OutDataTypeStr=boolean  RndMeth=Simplest
  Out1 : Outport
  wires:
  Data Type Conversion3/1 -> MinMax4/1
  Data Type Conversion1/1 -> MinMax2/1
  Data Type Conversion/1 -> MinMax1/1
  MinMax1/1 -> Memory1/1, MinMax/1
  ROOut4/1 -> Data Type Conversion3/1
  MinMax2/1 -> Memory2/1, MinMax/2
  ROOut1/1 -> Data Type Conversion/1
  Memory2/1 -> MinMax2/2
  Memory4/1 -> MinMax4/2
  ROOut2/1 -> Data Type Conversion1/1
  MinMax4/1 -> Memory4/1, MinMax/4
  Memory1/1 -> MinMax1/2
  [out4] -> ROOut4/2
  In4/1 -> ROOut4/1
  [out2] -> ROOut2/2
  In1/1 -> ROOut1/1
  In2/1 -> ROOut2/1
  [out1] -> ROOut1/2
  MinMax/1 -> Out1/1
  Constant3/1 -> MinMax/3

== system c00014M_harness/Eval33 ==
  In1 : Inport
  In2 : Inport  Port=2
  In4 : Inport  Port=3
  Constant3 : Constant
  Data Type Conversion : DataTypeConversion
  Data Type Conversion1 : DataTypeConversion
  Data Type Conversion3 : DataTypeConversion
  Memory1 : Memory  InitialCondition=1
  Memory2 : Memory  InitialCondition=1
  Memory4 : Memory  InitialCondition=1
  MinMax : MinMax  Inputs=4
  MinMax1 : MinMax  Inputs=2
  MinMax2 : MinMax  Inputs=2
  MinMax4 : MinMax  Inputs=2
  ROOut1 : RelationalOperator  Operator===  OutDataTypeStr=boolean  RndMeth=Simplest
  ROOut2 : RelationalOperator  Operator===  OutDataTypeStr=boolean  RndMeth=Simplest
  ROOut4 : RelationalOperator  Operator===  OutDataTypeStr=boolean  RndMeth=Simplest
  Out1 : Outport
  wires:
  Data Type Conversion3/1 -> MinMax4/1
  Data Type Conversion1/1 -> MinMax2/1
  Data Type Conversion/1 -> MinMax1/1
  MinMax1/1 -> Memory1/1, MinMax/1
  ROOut4/1 -> Data Type Conversion3/1
  MinMax2/1 -> Memory2/1, MinMax/2
  ROOut1/1 -> Data Type Conversion/1
  Memory2/1 -> MinMax2/2
  Memory4/1 -> MinMax4/2
  ROOut2/1 -> Data Type Conversion1/1
  MinMax4/1 -> Memory4/1, MinMax/4
  Memory1/1 -> MinMax1/2
  [out4] -> ROOut4/2
  In4/1 -> ROOut4/1
  [out2] -> ROOut2/2
  In1/1 -> ROOut1/1
  In2/1 -> ROOut2/1
  [out1] -> ROOut1/2
  MinMax/1 -> Out1/1
  Constant3/1 -> MinMax/3

== system c00014M_harness/Eval4 ==
  In1 : Inport
  In2 : Inport  Port=2
  In4 : Inport  Port=3
  Constant3 : Constant
  Data Type Conversion : DataTypeConversion
  Data Type Conversion1 : DataTypeConversion
  Data Type Conversion3 : DataTypeConversion
  Memory1 : Memory  InitialCondition=1
  Memory2 : Memory  InitialCondition=1
  Memory4 : Memory  InitialCondition=1
  MinMax : MinMax  Inputs=4
  MinMax1 : MinMax  Inputs=2
  MinMax2 : MinMax  Inputs=2
  MinMax4 : MinMax  Inputs=2
  ROOut1 : RelationalOperator  Operator===  OutDataTypeStr=boolean  RndMeth=Simplest
  ROOut2 : RelationalOperator  Operator===  OutDataTypeStr=boolean  RndMeth=Simplest
  ROOut4 : RelationalOperator  Operator===  OutDataTypeStr=boolean  RndMeth=Simplest
  Out1 : Outport
  wires:
  Data Type Conversion3/1 -> MinMax4/1
  Data Type Conversion1/1 -> MinMax2/1
  Data Type Conversion/1 -> MinMax1/1
  MinMax1/1 -> Memory1/1, MinMax/1
  ROOut4/1 -> Data Type Conversion3/1
  MinMax2/1 -> Memory2/1, MinMax/2
  ROOut1/1 -> Data Type Conversion/1
  Memory2/1 -> MinMax2/2
  Memory4/1 -> MinMax4/2
  ROOut2/1 -> Data Type Conversion1/1
  MinMax4/1 -> Memory4/1, MinMax/4
  Memory1/1 -> MinMax1/2
  [out4] -> ROOut4/2
  In4/1 -> ROOut4/1
  [out2] -> ROOut2/2
  In1/1 -> ROOut1/1
  In2/1 -> ROOut2/1
  [out1] -> ROOut1/2
  MinMax/1 -> Out1/1
  Constant3/1 -> MinMax/3

== system c00014M_harness/Eval43 ==
  In1 : Inport
  In2 : Inport  Port=2
  In4 : Inport  Port=3
  Constant3 : Constant
  Data Type Conversion : DataTypeConversion
  Data Type Conversion1 : DataTypeConversion
  Data Type Conversion3 : DataTypeConversion
  Memory1 : Memory  InitialCondition=1
  Memory2 : Memory  InitialCondition=1
  Memory4 : Memory  InitialCondition=1
  MinMax : MinMax  Inputs=4
  MinMax1 : MinMax  Inputs=2
  MinMax2 : MinMax  Inputs=2
  MinMax4 : MinMax  Inputs=2
  ROOut1 : RelationalOperator  Operator===  OutDataTypeStr=boolean  RndMeth=Simplest
  ROOut2 : RelationalOperator  Operator===  OutDataTypeStr=boolean  RndMeth=Simplest
  ROOut4 : RelationalOperator  Operator===  OutDataTypeStr=boolean  RndMeth=Simplest
  Out1 : Outport
  wires:
  Data Type Conversion3/1 -> MinMax4/1
  Data Type Conversion1/1 -> MinMax2/1
  Data Type Conversion/1 -> MinMax1/1
  MinMax1/1 -> Memory1/1, MinMax/1
  ROOut4/1 -> Data Type Conversion3/1
  MinMax2/1 -> Memory2/1, MinMax/2
  ROOut1/1 -> Data Type Conversion/1
  Memory2/1 -> MinMax2/2
  Memory4/1 -> MinMax4/2
  ROOut2/1 -> Data Type Conversion1/1
  MinMax4/1 -> Memory4/1, MinMax/4
  Memory1/1 -> MinMax1/2
  [out4] -> ROOut4/2
  In4/1 -> ROOut4/1
  [out2] -> ROOut2/2
  In1/1 -> ROOut1/1
  In2/1 -> ROOut2/1
  [out1] -> ROOut1/2
  MinMax/1 -> Out1/1
  Constant3/1 -> MinMax/3

== system c00014M_harness/Eval45 ==
  In1 : Inport
  In2 : Inport  Port=2
  In4 : Inport  Port=3
  Constant3 : Constant
  Data Type Conversion : DataTypeConversion
  Data Type Conversion1 : DataTypeConversion
  Data Type Conversion3 : DataTypeConversion
  Memory1 : Memory  InitialCondition=1
  Memory2 : Memory  InitialCondition=1
  Memory4 : Memory  InitialCondition=1
  MinMax : MinMax  Inputs=4
  MinMax1 : MinMax  Inputs=2
  MinMax2 : MinMax  Inputs=2
  MinMax4 : MinMax  Inputs=2
  ROOut1 : RelationalOperator  Operator===  OutDataTypeStr=boolean  RndMeth=Simplest
  ROOut2 : RelationalOperator  Operator===  OutDataTypeStr=boolean  RndMeth=Simplest
  ROOut4 : RelationalOperator  Operator===  OutDataTypeStr=boolean  RndMeth=Simplest
  Out1 : Outport
  wires:
  Data Type Conversion3/1 -> MinMax4/1
  Data Type Conversion1/1 -> MinMax2/1
  Data Type Conversion/1 -> MinMax1/1
  MinMax1/1 -> Memory1/1, MinMax/1
  ROOut4/1 -> Data Type Conversion3/1
  MinMax2/1 -> Memory2/1, MinMax/2
  ROOut1/1 -> Data Type Conversion/1
  Memory2/1 -> MinMax2/2
  Memory4/1 -> MinMax4/2
  ROOut2/1 -> Data Type Conversion1/1
  MinMax4/1 -> Memory4/1, MinMax/4
  Memory1/1 -> MinMax1/2
  [out4] -> ROOut4/2
  In4/1 -> ROOut4/1
  [out2] -> ROOut2/2
  In1/1 -> ROOut1/1
  In2/1 -> ROOut2/1
  [out1] -> ROOut1/2
  MinMax/1 -> Out1/1
  Constant3/1 -> MinMax/3

== system c00014M_harness/Eval47 ==
  In1 : Inport
  In2 : Inport  Port=2
  In4 : Inport  Port=3
  Constant3 : Constant
  Data Type Conversion : DataTypeConversion
  Data Type Conversion1 : DataTypeConversion
  Data Type Conversion3 : DataTypeConversion
  Memory1 : Memory  InitialCondition=1
  Memory2 : Memory  InitialCondition=1
  Memory4 : Memory  InitialCondition=1
  MinMax : MinMax  Inputs=4
  MinMax1 : MinMax  Inputs=2
  MinMax2 : MinMax  Inputs=2
  MinMax4 : MinMax  Inputs=2
  ROOut1 : RelationalOperator  Operator===  OutDataTypeStr=boolean  RndMeth=Simplest
  ROOut2 : RelationalOperator  Operator===  OutDataTypeStr=boolean  RndMeth=Simplest
  ROOut4 : RelationalOperator  Operator===  OutDataTypeStr=boolean  RndMeth=Simplest
  Out1 : Outport
  wires:
  Data Type Conversion3/1 -> MinMax4/1
  Data Type Conversion1/1 -> MinMax2/1
  Data Type Conversion/1 -> MinMax1/1
  MinMax1/1 -> Memory1/1, MinMax/1
  ROOut4/1 -> Data Type Conversion3/1
  MinMax2/1 -> Memory2/1, MinMax/2
  ROOut1/1 -> Data Type Conversion/1
  Memory2/1 -> MinMax2/2
  Memory4/1 -> MinMax4/2
  ROOut2/1 -> Data Type Conversion1/1
  MinMax4/1 -> Memory4/1, MinMax/4
  Memory1/1 -> MinMax1/2
  [out4] -> ROOut4/2
  In4/1 -> ROOut4/1
  [out2] -> ROOut2/2
  In1/1 -> ROOut1/1
  In2/1 -> ROOut2/1
  [out1] -> ROOut1/2
  MinMax/1 -> Out1/1
  Constant3/1 -> MinMax/3

== system c00014M_harness/Eval49 ==
  In1 : Inport
  In2 : Inport  Port=2
  In4 : Inport  Port=3
  Constant3 : Constant
  Data Type Conversion : DataTypeConversion
  Data Type Conversion1 : DataTypeConversion
  Data Type Conversion3 : DataTypeConversion
  Memory1 : Memory  InitialCondition=1
  Memory2 : Memory  InitialCondition=1
  Memory4 : Memory  InitialCondition=1
  MinMax : MinMax  Inputs=4
  MinMax1 : MinMax  Inputs=2
  MinMax2 : MinMax  Inputs=2
  MinMax4 : MinMax  Inputs=2
  ROOut1 : RelationalOperator  Operator===  OutDataTypeStr=boolean  RndMeth=Simplest
  ROOut2 : RelationalOperator  Operator===  OutDataTypeStr=boolean  RndMeth=Simplest
  ROOut4 : RelationalOperator  Operator===  OutDataTypeStr=boolean  RndMeth=Simplest
  Out1 : Outport
  wires:
  Data Type Conversion3/1 -> MinMax4/1
  Data Type Conversion1/1 -> MinMax2/1
  Data Type Conversion/1 -> MinMax1/1
  MinMax1/1 -> Memory1/1, MinMax/1
  ROOut4/1 -> Data Type Conversion3/1
  MinMax2/1 -> Memory2/1, MinMax/2
  ROOut1/1 -> Data Type Conversion/1
  Memory2/1 -> MinMax2/2
  Memory4/1 -> MinMax4/2
  ROOut2/1 -> Data Type Conversion1/1
  MinMax4/1 -> Memory4/1, MinMax/4
  Memory1/1 -> MinMax1/2
  [out4] -> ROOut4/2
  In4/1 -> ROOut4/1
  [out2] -> ROOut2/2
  In1/1 -> ROOut1/1
  In2/1 -> ROOut2/1
  [out1] -> ROOut1/2
  MinMax/1 -> Out1/1
  Constant3/1 -> MinMax/3

== system c00014M_harness/Eval50 ==
  In1 : Inport
  In2 : Inport  Port=2
  In4 : Inport  Port=3
  Constant3 : Constant
  Data Type Conversion : DataTypeConversion
  Data Type Conversion1 : DataTypeConversion
  Data Type Conversion3 : DataTypeConversion
  Memory1 : Memory  InitialCondition=1
  Memory2 : Memory  InitialCondition=1
  Memory4 : Memory  InitialCondition=1
  MinMax : MinMax  Inputs=4
  MinMax1 : MinMax  Inputs=2
  MinMax2 : MinMax  Inputs=2
  MinMax4 : MinMax  Inputs=2
  ROOut1 : RelationalOperator  Operator===  OutDataTypeStr=boolean  RndMeth=Simplest
  ROOut2 : RelationalOperator  Operator===  OutDataTypeStr=boolean  RndMeth=Simplest
  ROOut4 : RelationalOperator  Operator===  OutDataTypeStr=boolean  RndMeth=Simplest
  Out1 : Outport
  wires:
  Data Type Conversion3/1 -> MinMax4/1
  Data Type Conversion1/1 -> MinMax2/1
  Data Type Conversion/1 -> MinMax1/1
  MinMax1/1 -> Memory1/1, MinMax/1
  ROOut4/1 -> Data Type Conversion3/1
  MinMax2/1 -> Memory2/1, MinMax/2
  ROOut1/1 -> Data Type Conversion/1
  Memory2/1 -> MinMax2/2
  Memory4/1 -> MinMax4/2
  ROOut2/1 -> Data Type Conversion1/1
  MinMax4/1 -> Memory4/1, MinMax/4
  Memory1/1 -> MinMax1/2
  [out4] -> ROOut4/2
  In4/1 -> ROOut4/1
  [out2] -> ROOut2/2
  In1/1 -> ROOut1/1
  In2/1 -> ROOut2/1
  [out1] -> ROOut1/2
  MinMax/1 -> Out1/1
  Constant3/1 -> MinMax/3

== system c00014M_harness/Eval51 ==
  In1 : Inport
  In2 : Inport  Port=2
  In4 : Inport  Port=3
  Constant3 : Constant
  Data Type Conversion : DataTypeConversion
  Data Type Conversion1 : DataTypeConversion
  Data Type Conversion3 : DataTypeConversion
  Memory1 : Memory  InitialCondition=1
  Memory2 : Memory  InitialCondition=1
  Memory4 : Memory  InitialCondition=1
  MinMax : MinMax  Inputs=4
  MinMax1 : MinMax  Inputs=2
  MinMax2 : MinMax  Inputs=2
  MinMax4 : MinMax  Inputs=2
  ROOut1 : RelationalOperator  Operator===  OutDataTypeStr=boolean  RndMeth=Simplest
  ROOut2 : RelationalOperator  Operator===  OutDataTypeStr=boolean  RndMeth=Simplest
  ROOut4 : RelationalOperator  Operator===  OutDataTypeStr=boolean  RndMeth=Simplest
  Out1 : Outport
  wires:
  Data Type Conversion3/1 -> MinMax4/1
  Data Type Conversion1/1 -> MinMax2/1
  Data Type Conversion/1 -> MinMax1/1
  MinMax1/1 -> Memory1/1, MinMax/1
  ROOut4/1 -> Data Type Conversion3/1
  MinMax2/1 -> Memory2/1, MinMax/2
  ROOut1/1 -> Data Type Conversion/1
  Memory2/1 -> MinMax2/2
  Memory4/1 -> MinMax4/2
  ROOut2/1 -> Data Type Conversion1/1
  MinMax4/1 -> Memory4/1, MinMax/4
  Memory1/1 -> MinMax1/2
  [out4] -> ROOut4/2
  In4/1 -> ROOut4/1
  [out2] -> ROOut2/2
  In1/1 -> ROOut1/1
  In2/1 -> ROOut2/1
  [out1] -> ROOut1/2
  MinMax/1 -> Out1/1
  Constant3/1 -> MinMax/3

== system c00014M_harness/Eval55 ==
  In1 : Inport
  In2 : Inport  Port=2
  In4 : Inport  Port=3
  Constant3 : Constant
  Data Type Conversion : DataTypeConversion
  Data Type Conversion1 : DataTypeConversion
  Data Type Conversion3 : DataTypeConversion
  Memory1 : Memory  InitialCondition=1
  Memory2 : Memory  InitialCondition=1
  Memory4 : Memory  InitialCondition=1
  MinMax : MinMax  Inputs=4
  MinMax1 : MinMax  Inputs=2
  MinMax2 : MinMax  Inputs=2
  MinMax4 : MinMax  Inputs=2
  ROOut1 : RelationalOperator  Operator===  OutDataTypeStr=boolean  RndMeth=Simplest
  ROOut2 : RelationalOperator  Operator===  OutDataTypeStr=boolean  RndMeth=Simplest
  ROOut4 : RelationalOperator  Operator===  OutDataTypeStr=boolean  RndMeth=Simplest
  Out1 : Outport
  wires:
  Data Type Conversion3/1 -> MinMax4/1
  Data Type Conversion1/1 -> MinMax2/1
  Data Type Conversion/1 -> MinMax1/1
  MinMax1/1 -> Memory1/1, MinMax/1
  ROOut4/1 -> Data Type Conversion3/1
  MinMax2/1 -> Memory2/1, MinMax/2
  ROOut1/1 -> Data Type Conversion/1
  Memory2/1 -> MinMax2/2
  Memory4/1 -> MinMax4/2
  ROOut2/1 -> Data Type Conversion1/1
  MinMax4/1 -> Memory4/1, MinMax/4
  Memory1/1 -> MinMax1/2
  [out4] -> ROOut4/2
  In4/1 -> ROOut4/1
  [out2] -> ROOut2/2
  In1/1 -> ROOut1/1
  In2/1 -> ROOut2/1
  [out1] -> ROOut1/2
  MinMax/1 -> Out1/1
  Constant3/1 -> MinMax/3

== system c00014M_harness/Inputs ==
  Demux : Demux  Tag=STV Demux  Outputs=13
  FromWs : FromWorkspace  Tag=STV FromWs  VariableName=tuvar  SampleTime=0
  DW1 : Outport  Tag=STV Outport
  DW2 : Outport  Tag=STV Outport  Port=2
  DW4 : Outport  Tag=STV Outport  Port=3
  P1W2 : Outport  Tag=STV Outport  Port=4
  P3W4 : Outport  Tag=STV Outport  Port=5
  P1W4 : Outport  Tag=STV Outport  Port=6
  O1 : Outport  Tag=STV Outport  Port=7
  O2 : Outport  Tag=STV Outport  Port=8
  O4 : Outport  Tag=STV Outport  Port=9
  LD : Outport  Tag=STV Outport  Port=10
  CW1C : Outport  Tag=STV Outport  Port=11
  CW2C : Outport  Tag=STV Outport  Port=12
  CW4C : Outport  Tag=STV Outport  Port=13
  wires:
  Demux/13 -> CW4C/1
  Demux/12 -> CW2C/1
  Demux/11 -> CW1C/1
  Demux/10 -> LD/1
  Demux/9 -> O4/1
  Demux/8 -> O2/1
  Demux/7 -> O1/1
  Demux/6 -> P1W4/1
  Demux/5 -> P3W4/1
  Demux/4 -> P1W2/1
  Demux/3 -> DW4/1
  Demux/2 -> DW2/1
  Demux/1 -> DW1/1
  FromWs/1 -> Demux/1

== system c00014M_harness/M001 ==
  DW1 : Inport  OutMin=0  OutMax=4  OutDataTypeStr=int8
  DW2 : Inport  Port=2  OutMin=0  OutMax=4  OutDataTypeStr=int8
  DW4 : Inport  Port=3  OutMin=0  OutMax=4  OutDataTypeStr=int8
  P1W2 : Inport  Port=4  OutMin=0  OutMax=4  OutDataTypeStr=int8
  P3W4 : Inport  Port=5  OutMin=0  OutMax=4  OutDataTypeStr=int8
  P1W4 : Inport  Port=6  OutMin=0  OutMax=4  OutDataTypeStr=int8
  O1 : Inport  Port=7  OutDataTypeStr=boolean
  O2 : Inport  Port=8  OutDataTypeStr=boolean
  O4 : Inport  Port=9  OutDataTypeStr=boolean
  LD : Inport  Port=10  OutDataTypeStr=boolean
  CW1C : Inport  Port=11  OutMin=0  OutMax=4  OutDataTypeStr=int8
  CW2C : Inport  Port=12  OutMin=0  OutMax=4  OutDataTypeStr=int8
  CW4C : Inport  Port=13  OutMin=0  OutMax=4  OutDataTypeStr=int8
  Cyber : Subsystem
  M : Memory
  M1 : Memory
  M3 : Memory
  Physical : Subsystem
  S1 : Subsystem
  S2 : Subsystem
  S4 : Subsystem
  W1Pos : Outport
  W2Pos : Outport  Port=2
  W4Pos : Outport  Port=3
  wires:
  M3/1 -> Cyber/3(PosW4)
  S1/1(SensorOut) -> M/1
  CW2C/1 -> Cyber/15(CW2C)
  CW4C/1 -> Cyber/16(CW4C)
  Physical/1(W1) -> W1Pos/1, S1/1(PhyMeasure)
  O4/1 -> Cyber/12(OW4)
  O2/1 -> Cyber/11(OW2)
  LD/1 -> Cyber/13(LD)
  O1/1 -> Cyber/10(OW1)
  Cyber/1(W1) -> Physical/1(InW1)
  Cyber/2(W2) -> Physical/2(InW2)
  P1W2/1 -> Cyber/7(P1W2)
  P1W4/1 -> Cyber/9(P1W4)
  CW1C/1 -> Cyber/14(CW1C)
  S4/1(SensorOut) -> M3/1
  M1/1 -> Cyber/2(PosW2)
  M/1 -> Cyber/1(PosW1)
  DW1/1 -> Cyber/4(DW1)
  Physical/2(W2) -> W2Pos/1, S2/1(PhyMeasure)
  S2/1(SensorOut) -> M1/1
  P3W4/1 -> Cyber/8(P3W4)
  DW2/1 -> Cyber/5(DW2)
  Physical/3(W4) -> W4Pos/1, S4/1(PhyMeasure)
  DW4/1 -> Cyber/6(DW4)
  Cyber/3(W4) -> Physical/3(InW4)

== system c00014M_harness/M003 ==
  DW1 : Inport  OutMin=0  OutMax=4  OutDataTypeStr=int8
  DW2 : Inport  Port=2  OutMin=0  OutMax=4  OutDataTypeStr=int8
  DW4 : Inport  Port=3  OutMin=0  OutMax=4  OutDataTypeStr=int8
  P1W2 : Inport  Port=4  OutMin=0  OutMax=4  OutDataTypeStr=int8
  P3W4 : Inport  Port=5  OutMin=0  OutMax=4  OutDataTypeStr=int8
  P1W4 : Inport  Port=6  OutMin=0  OutMax=4  OutDataTypeStr=int8
  O1 : Inport  Port=7  OutDataTypeStr=boolean
  O2 : Inport  Port=8  OutDataTypeStr=boolean
  O4 : Inport  Port=9  OutDataTypeStr=boolean
  LD : Inport  Port=10  OutDataTypeStr=boolean
  CW1C : Inport  Port=11  OutMin=0  OutMax=4  OutDataTypeStr=int8
  CW2C : Inport  Port=12  OutMin=0  OutMax=4  OutDataTypeStr=int8
  CW4C : Inport  Port=13  OutMin=0  OutMax=4  OutDataTypeStr=int8
  Cyber : Subsystem
  M : Memory
  M1 : Memory
  M3 : Memory
  Physical : Subsystem
  S1 : Subsystem
  S2 : Subsystem
  S4 : Subsystem
  W1Pos : Outport
  W2Pos : Outport  Port=2
  W4Pos : Outport  Port=3
  wires:
  Cyber/3(W4) -> Physical/3(InW4)
  DW4/1 -> Cyber/6(DW4)
  Physical/3(W4) -> S4/1(PhyMeasure), W4Pos/1
  DW2/1 -> Cyber/5(DW2)
  P3W4/1 -> Cyber/8(P3W4)
  S2/1(SensorOut) -> M1/1
  Physical/2(W2) -> S2/1(PhyMeasure), W2Pos/1
  DW1/1 -> Cyber/4(DW1)
  M/1 -> Cyber/1(PosW1)
  M1/1 -> Cyber/2(PosW2)
  S4/1(SensorOut) -> M3/1
  CW1C/1 -> Cyber/14(CW1C)
  P1W4/1 -> Cyber/9(P1W4)
  P1W2/1 -> Cyber/7(P1W2)
  Cyber/2(W2) -> Physical/2(InW2)
  Cyber/1(W1) -> Physical/1(InW1)
  O1/1 -> Cyber/10(OW1)
  LD/1 -> Cyber/13(LD)
  O2/1 -> Cyber/11(OW2)
  O4/1 -> Cyber/12(OW4)
  Physical/1(W1) -> S1/1(PhyMeasure), W1Pos/1
  CW4C/1 -> Cyber/16(CW4C)
  CW2C/1 -> Cyber/15(CW2C)
  S1/1(SensorOut) -> M/1
  M3/1 -> Cyber/3(PosW4)

== system c00014M_harness/M005 ==
  DW1 : Inport  OutMin=0  OutMax=4  OutDataTypeStr=int8
  DW2 : Inport  Port=2  OutMin=0  OutMax=4  OutDataTypeStr=int8
  DW4 : Inport  Port=3  OutMin=0  OutMax=4  OutDataTypeStr=int8
  P1W2 : Inport  Port=4  OutMin=0  OutMax=4  OutDataTypeStr=int8
  P3W4 : Inport  Port=5  OutMin=0  OutMax=4  OutDataTypeStr=int8
  P1W4 : Inport  Port=6  OutMin=0  OutMax=4  OutDataTypeStr=int8
  O1 : Inport  Port=7  OutDataTypeStr=boolean
  O2 : Inport  Port=8  OutDataTypeStr=boolean
  O4 : Inport  Port=9  OutDataTypeStr=boolean
  LD : Inport  Port=10  OutDataTypeStr=boolean
  CW1C : Inport  Port=11  OutMin=0  OutMax=4  OutDataTypeStr=int8
  CW2C : Inport  Port=12  OutMin=0  OutMax=4  OutDataTypeStr=int8
  CW4C : Inport  Port=13  OutMin=0  OutMax=4  OutDataTypeStr=int8
  Cyber : Subsystem
  M : Memory
  M1 : Memory
  M3 : Memory
  Physical : Subsystem
  S1 : Subsystem
  S2 : Subsystem
  S4 : Subsystem
  W1Pos : Outport
  W2Pos : Outport  Port=2
  W4Pos : Outport  Port=3
  wires:
  Cyber/3(W4) -> Physical/3(InW4)
  DW4/1 -> Cyber/6(DW4)
  Physical/3(W4) -> S4/1(PhyMeasure), W4Pos/1
  DW2/1 -> Cyber/5(DW2)
  P3W4/1 -> Cyber/8(P3W4)
  S2/1(SensorOut) -> M1/1
  Physical/2(W2) -> S2/1(PhyMeasure), W2Pos/1
  DW1/1 -> Cyber/4(DW1)
  M/1 -> Cyber/1(PosW1)
  M1/1 -> Cyber/2(PosW2)
  S4/1(SensorOut) -> M3/1
  CW1C/1 -> Cyber/14(CW1C)
  P1W4/1 -> Cyber/9(P1W4)
  P1W2/1 -> Cyber/7(P1W2)
  Cyber/2(W2) -> Physical/2(InW2)
  Cyber/1(W1) -> Physical/1(InW1)
  O1/1 -> Cyber/10(OW1)
  LD/1 -> Cyber/13(LD)
  O2/1 -> Cyber/11(OW2)
  O4/1 -> Cyber/12(OW4)
  Physical/1(W1) -> S1/1(PhyMeasure), W1Pos/1
  CW4C/1 -> Cyber/16(CW4C)
  CW2C/1 -> Cyber/15(CW2C)
  S1/1(SensorOut) -> M/1
  M3/1 -> Cyber/3(PosW4)
